simulink library "vmc"  (R2021b)
settings: Solver=VariableStepAuto  StartTime=0.0  StopTime=10.0  RelTol=1e-3
undefined symbols (not defined in the file or in its folder): AVMC_ACCDeltaTqIGain_X_kph, AVMC_ACCDeltaTqIGain_Y_mps2, AVMC_ACCDeltaTqPGain_X_kph, AVMC_ACCDeltaTqPGain_Y_kph, AVMC_ACCLongSteadyCtrl_X_kph, AVMC_AggressJerkPCT4AT_X_kph, AVMC_AggressJerkPCT_X_kph, AVMC_AggressLimitPCT4AT_X_kph, AVMC_AggressLimitPCT_X_kph, AVMC_CCLongSteadyCtrl_X_kph, AVMC_DISCDeltaTqIGain_X_kph, AVMC_DISCDeltaTqIGain_Y_mps2, AVMC_DISCDeltaTqPGain_X_kph, AVMC_DISCDeltaTqPGain_Y_kph, AVMC_DISCTrunAccJerk_X_s, AVMC_DISCTrunAccLimit_X_s, AVMC_ESCRegenOut_X_kph, AVMC_ESCRegenOut_Y_Deg, AVMC_ESCRegenOutEnSpd_X_Deg, AVMC_ISOAccLimit_X_mps, AVMC_ISODecLimit_X_mps, AVMC_ISOJerk_X_mps, AVMC_LatESCRegenOut_X_kph, AVMC_LatESCRegenOut_Y_Deg, AVMC_LongAccDeadZone_X_kph, AVMC_LongAccFiltTsforP2_X_Gps, AVMC_MCPresBaseTq_X_bar, AVMC_MSALongSteadyCtrl_X_kph, AVMC_MSAPedalOvrd2_X_kph, AVMC_MSAPedalOvrd_X_kph, AVMC_MSASpdBand_X_kph, AVMC_MSATqDownEndTq_X_kph, AVMC_MSATqDownTime_X_kph, AVMC_OPDDisSlideRate_X_Deg, AVMC_RDCDetectTime_X_kph, AVMC_RDCDetectTime_Y_pct, AVMC_RDCEnSlideRate_X_Deg, AVMC_RearWhlTqRatio_X_Nm, AVMC_RearWhlTqRatio_Y_gps, AVMC_RearWhlTqSlipGain_X_rat, AVMC_RearWhlTqSlipGain_Y_kph, AVMC_RearWhlTqSTRGGain_X_deg, AVMC_RearWhlTqSTRGGain_Y_kph, AVMC_RWSRrTSA2RWSPos_X_deg, AVMC_RWSSAS2FrtTSA_X_deg, AVMC_RWSVehSPD2RWSCoef_X_kph, AVMC_SoftJerkPCT_X_kph, AVMC_SoftLimitPCT_X_kph, AVMC_StESCYaw_X_kph, AVMC_StESCYaw_Y_Deg, AVMC_StESCYawCom_X_kph, AVMC_StESCYawCom_Y_Gps, AVMC_TMSpdBaseTq_X_rpm, AVMC_VehHoldBDecMap_X_kph, AVMC_VehHoldDecCtrlTime_X_kph, AVMC_VehHoldMCPPass_X_deg, C_TASK_10MS_S, C_TASK_5MS_S, DEG2RAD, ENUM_ACCAVAIL_AVAILABLE ... (+409)
libraries: hcu_lib x74, simulink x68, simulink_extras x3, $bdroot x2
(part 1 of 15)
settings Model: Creator=FVT22120  LastModifiedBy=FVT23010

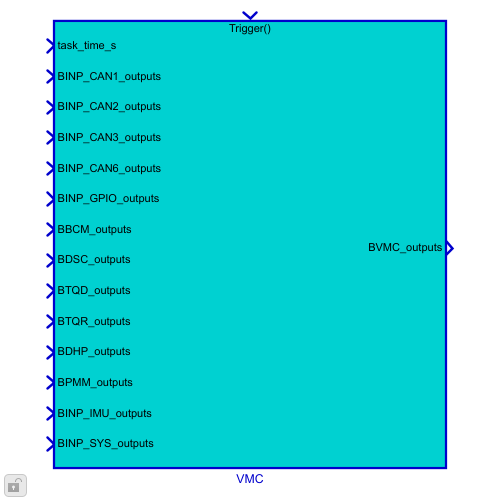
[thumbnail: Simulink's stored preview of the top-level diagram]
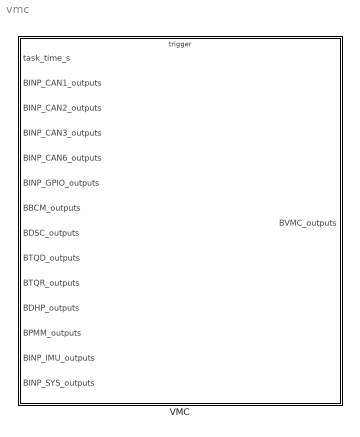
== system vmc ==
  VMC : Subsystem
      settings: RTWSystemCode=Nonreusable function  RTWFcnNameOpts=Use subsystem name  RTWFileNameOpts=Use subsystem name

== system vmc/VMC ==
  task_time_s : Inport
  BINP_CAN1_outputs : Inport  Port=2  OutDataTypeStr=Bus: BINP_CAN1_outputs
  BINP_CAN2_outputs : Inport  Port=3  OutDataTypeStr=Bus: BINP_CAN2_outputs
  BINP_CAN3_outputs : Inport  Port=4  OutDataTypeStr=Bus: BINP_CAN3_outputs
  BINP_CAN6_outputs : Inport  Port=5  OutDataTypeStr=Bus: BINP_CAN6_outputs
  BINP_GPIO_outputs : Inport  Port=6  OutDataTypeStr=Bus: BINP_GPIO_outputs
  BBCM_outputs : Inport  Port=7  OutDataTypeStr=Bus: BBCM_outputs
  BDSC_outputs : Inport  Port=8  OutDataTypeStr=Bus: BDSC_outputs
  BTQD_outputs : Inport  Port=9  OutDataTypeStr=Bus: BTQD_outputs
  BTQR_outputs : Inport  Port=10  OutDataTypeStr=Bus: BTQR_outputs
  BDHP_outputs : Inport  Port=11  OutDataTypeStr=Bus: BDHP_outputs
  BPMM_outputs : Inport  Port=12  OutDataTypeStr=Bus: BPMM_outputs
  BINP_IMU_outputs : Inport  Port=13  OutDataTypeStr=Bus: BINP_IMU_outputs
  BINP_SYS_outputs : Inport  Port=14  OutDataTypeStr=Bus: BINP_SYS_outputs
  Trigger : TriggerPort  TriggerType=function-call  VariantControl=(inherit)  PortDimensions=1
  Bus Creator1 : BusCreator  Inputs=148  OutDataTypeStr=Bus: BVMC_outputs  NonVirtualBus=on
  Bus Selector : BusSelector  OutputSignals=VINP_DriverSeatBeltCmd_flg,VINP_MeterIndVehSpeed_kph,VINP_BrkSwSta_flg,VINP_EPBSta_enum,VINP_ACCAvail_flg,VINP_AEBAvail_flg,VINP_ESCOFFStatus_enum,VINP_VehSpeed_kph,VINP_LFRawWhlSpeed_kph,VINP_LFRawWhlSpeedV_flg,VINP_RFRawWhlSpeed_kph,VINP_RFRawWhlSpeedV_flg,VINP_LRRawWhlSpeed_kph,VINP_LRRawWhlSpeedV_flg,VINP_RRRawWhlSpeed_kph,VINP_RRRawWhlSpeedV_flg,VINP_LatAccel_Gps,VINP_LatAccelV_flg,VINP_GRADE_Deg,VINP_LongAccel_Gps,VINP_MCPressure_bar,VINP_ESCADASSta_enum,VINP_FrRBCActive_flg,VINP_RrRBCActive_flg,VINP_FrntAxlTrqReqBrk_Nm,VINP_RearAxlTrqReqBrk_Nm,VINP_BrkPedalPos_pct,VINP_SASAngle_Deg,VINP_ESCActive_flg,VINP_YawRate_degps,VINP_RDCActive_enum,VINP_LFWhlRotDir_enum,VINP_LRWhlRotDir_enum,VINP_RFWhlRotDir_enum,VINP_RRWhlRotDir_enum
  Bus Selector10 : BusSelector  OutputSignals=VDHP_ActAPSPosn_pct
  Bus Selector11 : BusSelector  OutputSignals=VPMM_DrivetrainSelect_enum
  Bus Selector12 : BusSelector  OutputSignals=VINP_DIDGetDynoMode_flg
  Bus Selector2 : BusSelector  OutputSignals=VBCM_DrDoorSW_flg
  Bus Selector3 : BusSelector  OutputSignals=VDSC_DISCTurn_flg,VDSC_DISCSta_enum,VDSC_DISCTargetSpd_kph
  Bus Selector4 : BusSelector  OutputSignals=VTQD_DriverWhlTqDem_Nm,VTQD_CoordWhlTqDemFr_Nm,VTQD_CoordWhlTqDemRr_Nm,VTQD_GearActualPosn_enum,VTQD_ExternalTqAllow_flg,VTQD_LowIdleAccPedal_flg,VTQD_ExtShftAllow_flg,VTQD_FrEDUAvailBrkRgnTq_Nm,VTQD_RrEDUAvailBrkRgnTq_Nm,VTQD_APSStaSys_enum,VTQD_APSDecReqA_flg,VTQD_APSDecReq_mps2,VTQD_APSReq_enum,VTQD_AfterAvailableTqDemFr_Nm,VTQD_AfterAvailableTqDemRr_Nm,VTQD_EquivAccPedalSWSta_flg,VTQD_ExtDoorAllow_flg,VTQD_SpdCtrlSta_flg,VTQD_SpdCtrlMode_enum,VTQD_RegenMode_enum,VTQD_SetSpd_kph,VTQD_SWCResUpSta_flg,VTQD_SWCSetdownSta_flg,VTQD_SWCCancelSta_flg,VTQD_CreepBaseTqD_Nm
  Bus Selector5 : BusSelector  OutputSignals=VINP_FrTMSpd_rpm,VINP_RrTMSpd_rpm
  Bus Selector6 : BusSelector  OutputSignals=VINP_BrakeSWGPIO_flg,VINP_HoodSW_flg
  Bus Selector7 : BusSelector  OutputSignals=VINP_ADASAEBSta_enum,VINP_ADASACCSta_enum,VINP_ACCRequiredAccel_mps2,VINP_ACCVehHoldReq_flg,VINP_ADASAEBReq_enum,VINP_ADASLKASta_enum,VINP_FCMLKAStrToqReq_Nm,VINP_FCMLKATOIFault_flg,VINP_FCMLKATOIAct_enum,VINP_ADASFaultSta_flg,VINP_AEBVehHoldReq_flg,VINP_ADASDBSReq_enum,VINP_ACCObjDist_m,VINP_ACCObjRelSpd_mps,VINP_TimeGapLevel_enum,VINP_HazardWarningReq_flg,VINP_ADASForceIdle_flg,VINP_RightTurnLightReq_flg,VINP_LeftTurnLightReq_flg,VINP_ForceLowBeam_enum,VINP_ACCJerkUpperLimit_mps3,VINP_ACCComfortBandUpper_mps2,VINP_ACCJerkLowerLimit_mps3,VINP_ACCComfortBandLower_mps2,VINP_ADASVehSpdLim_enum,VINP_ADASShftPosnReqA_flg,VINP_ADASShftPosnReq_enum,VINP_ADASFCWSta_enum,VINP_ADASLDWSta_enum,VINP_ADASFltWrnReq_flg,VINP_ACCObjDstLvl_enum,VINP_ACCTakeoverReq_flg,VINP_ADASWarningMsg_enum,VINP_ADASCAMSpdLim_enum,VINP_TargetType_enum,VINP_ADASSLIFSpdLim_enum,VINP_LKAHODDisplayWarning_flg,VINP_LKAHODSoundWarning_flg,VINP_ADASLFCSta_enum,VINP_ADASLaneModeL_enum,VINP_ADASLaneModeR_enum,VINP_ADASSLIFSta_enum,VINP_ADASISASta_enum,VINP_ADASLDWMute_flg,VINP_ADASFCWMute_flg,VINP_ADASLFCHandsOffWarning_enum,VINP_LVDADisabled_flg,VINP_LVDAMuteSta_enum,VINP_LVDAFailinfo_flg,VINP_LVDAWarning_flg,VINP_LVDAACCStatusInformation_flg,VINP_ADASLFCWarnSound_enum
  Bus Selector8 : BusSelector  OutputSignals=VINP_Distanceunit_flg,VINP_METERKPHCalcu_kph,VINP_GPSLAT_s,VINP_GPSLONG_enum
  Bus Selector9 : BusSelector  OutputSignals=VTQR_RrTMTqReq_Nm,VTQR_FrTMTqReq_Nm
  Ground{,1..20} (21 alike) : Ground
  VMC : Subsystem
  BVMC_outputs : Outport  OutDataTypeStr=Bus:BVMC_outputs
  wires:
  Bus Selector/24 -> VMC/25(VINP_RrRBCActive_flg)  "<VINP_RrRBCActive_flg>"
  Bus Selector/23 -> VMC/24(VINP_FrRBCActive_flg)  "<VINP_FrRBCActive_flg>"
  BINP_CAN3_outputs/1 -> Bus Selector5/1
  Bus Selector/22 -> VMC/23(VINP_ESCADASSta_enum)  "<VINP_ESCADASSta_enum>"
  Bus Selector/21 -> VMC/22(VINP_MCPressure_bar)  "<VINP_MCPressure_bar>"
  Bus Selector7/9 -> VMC/52(VINP_LKATOIAct_enum)  "<VINP_FCMLKATOIAct_enum>"
  Bus Selector7/8 -> VMC/51(VINP_LKATOIFault_flg)  "<VINP_FCMLKATOIFault_flg>"
  Bus Selector4/7 -> VMC/127(VTQD_ExtShftAllow_flg)  "<VTQD_ExtShftAllow_flg>"
  Bus Selector4/6 -> VMC/126(VTQD_LowIdleAccPedal_flg)  "<VTQD_LowIdleAccPedal_flg>"
  Bus Selector8/1 -> VMC/37(VINP_Distanceunit_flg)  "<VINP_Distanceunit_flg>"
  Bus Selector/1 -> VMC/2(VINP_DriverSeatBeltCmd_flg)  "<VINP_DriverSeatBeltCmd_flg>"
  Bus Selector7/15 -> VMC/58(VINP_TimeGapLevel_enum)  "<VINP_TimeGapLevel_enum>"
  Bus Selector7/14 -> VMC/57(VINP_ACCObjRelSpd_mps)  "<VINP_ACCObjRelSpd_mps>"
  Bus Selector7/13 -> VMC/56(VINP_ACCObjDist_m)  "<VINP_ACCObjDist_m>"
  Bus Selector7/12 -> VMC/55(VINP_ADASDBSReq_enum)  "<VINP_ADASDBSReq_enum>"
  Bus Selector7/11 -> VMC/54(VINP_AEBVehHoldReq_flg)  "<VINP_AEBVehHoldReq_flg>"
  Bus Selector7/10 -> VMC/53(VINP_ADASFaultSta_flg)  "<VINP_ADASFaultSta_flg>"
  Bus Selector7/7 -> VMC/50(VINP_LKAStrToqReq_Nm)  "<VINP_FCMLKAStrToqReq_Nm>"
  Bus Selector7/6 -> VMC/49(VINP_ADASLKASta_enum)  "<VINP_ADASLKASta_enum>"
  Bus Selector7/5 -> VMC/48(VINP_ADASAEBReq_enum)  "<VINP_ADASAEBReq_enum>"
  Bus Selector7/4 -> VMC/47(VINP_ACCVehHoldReq_flg)  "<VINP_ACCVehHoldReq_flg>"
  Bus Selector7/3 -> VMC/46(VINP_ACCRequiredAccel_mps2)  "<VINP_ACCRequiredAccel_mps2>"
  Bus Selector7/2 -> VMC/45(VINP_ADASACCSta_enum)  "<VINP_ADASACCSta_enum>"
  Bus Selector7/1 -> VMC/44(VINP_ADASAEBSta_enum)  "<VINP_ADASAEBSta_enum>"
  BINP_CAN6_outputs/1 -> Bus Selector7/1
  Bus Selector6/1 -> VMC/101(VINP_BrakeSWGPIO_flg)  "<VINP_BrakeSWGPIO_flg>"
  BINP_GPIO_outputs/1 -> Bus Selector6/1
  task_time_s/1 -> VMC/1(task_time_s)
  Bus Selector/9 -> VMC/10(VINP_LFRawWhlSpeed_kph)  "<VINP_LFRawWhlSpeed_kph>"
  Bus Selector/10 -> VMC/11(VINP_LFRawWhlSpeedV_flg)  "<VINP_LFRawWhlSpeedV_flg>"
  Bus Selector/11 -> VMC/12(VINP_RFRawWhlSpeed_kph)  "<VINP_RFRawWhlSpeed_kph>"
  Bus Selector/12 -> VMC/13(VINP_RFRawWhlSpeedV_flg)  "<VINP_RFRawWhlSpeedV_flg>"
  Bus Selector/13 -> VMC/14(VINP_LRRawWhlSpeed_kph)  "<VINP_LRRawWhlSpeed_kph>"
  Bus Selector/14 -> VMC/15(VINP_LRRawWhlSpeedV_flg)  "<VINP_LRRawWhlSpeedV_flg>"
  Bus Selector/15 -> VMC/16(VINP_RRRawWhlSpeed_kph)  "<VINP_RRRawWhlSpeed_kph>"
  Bus Selector/16 -> VMC/17(VINP_RRRawWhlSpeedV_flg)  "<VINP_RRRawWhlSpeedV_flg>"
  Bus Selector/17 -> VMC/18(VINP_LatAccel_Gps)  "<VINP_LatAccel_Gps>"
  Bus Selector/6 -> VMC/7(VINP_AEBAvail_flg)  "<VINP_AEBAvail_flg>"
  Bus Selector/18 -> VMC/19(VINP_LatAccelV_flg)  "<VINP_LatAccelV_flg>"
  Bus Selector/5 -> VMC/6(VINP_ACCAvail_flg)  "<VINP_ACCAvail_flg>"
  Bus Selector/19 -> VMC/20(VINP_GRADE_Deg)  "<VINP_GRADE_Deg>"
  Bus Selector/2 -> VMC/3(VINP_MeterIndVehSpeed_kph)  "<VINP_MeterIndVehSpeed_kph>"
  Bus Selector4/5 -> VMC/125(VTQD_ExternalTqAllow_flg)  "<VTQD_ExternalTqAllow_flg>"
  Bus Selector4/4 -> VMC/124(VTQD_GearActualPosn_enum)  "<VTQD_GearActualPosn_enum>"
  Bus Selector4/3 -> VMC/123(VTQD_CoordWhlTqDemRr_Nm)  "<VTQD_CoordWhlTqDemRr_Nm>"
  Bus Selector4/2 -> VMC/122(VTQD_CoordWhlTqDemFr_Nm)  "<VTQD_CoordWhlTqDemFr_Nm>"
  Bus Selector4/1 -> VMC/121(VTQD_DriverWhlTqDem_Nm)  "<VTQD_DriverWhlTqDem_Nm>"
  Bus Selector/20 -> VMC/21(VINP_LongAccel_Gps)  "<VINP_LongAccel_Gps>"
  Bus Selector/7 -> VMC/8(VINP_ESCOFFStatus_enum)  "<VINP_ESCOFFStatus_enum>"
  Bus Selector/8 -> VMC/9(VINP_VehSpeed_kph)  "<VINP_VehSpeed_kph>"
  Bus Selector/4 -> VMC/5(VINP_EPBSta_enum)  "<VINP_EPBSta_enum>"
  Bus Selector/3 -> VMC/4(VINP_BrkSwSta_flg)  "<VINP_BrkSwSta_flg>"
  BTQD_outputs/1 -> Bus Selector4/1
  Bus Selector3/3 -> VMC/117(VDSC_DISCTargetSpd_kph)  "<VDSC_DISCTargetSpd_kph>"
  Bus Selector3/2 -> VMC/116(VDSC_DISCSta_enum)  "<VDSC_DISCSta_enum>"
  Bus Selector3/1 -> VMC/115(VDSC_DISCTurn_flg)  "<VDSC_DISCTurn_flg>"
  BDSC_outputs/1 -> Bus Selector3/1
  Bus Selector2/1 -> VMC/114(VBCM_DrDoorSW_flg)  "<VBCM_DrDoorSW_flg>"
  BBCM_outputs/1 -> Bus Selector2/1
  BINP_CAN1_outputs/1 -> Bus Selector/1
  Bus Creator1/1 -> BVMC_outputs/1  "BVMC_outputs"
  Bus Selector/25 -> VMC/26(VINP_FrntAxlTrqReqBrk_Nm)  "<VINP_FrntAxlTrqReqBrk_Nm>"
  Bus Selector/26 -> VMC/27(VINP_RearAxlTrqReqBrk_Nm)  "<VINP_RearAxlTrqReqBrk_Nm>"
  Bus Selector7/16 -> VMC/59(VINP_HazardWarningReq_flg)  "<VINP_HazardWarningReq_flg>"
  BTQR_outputs/1 -> Bus Selector9/1
  Bus Selector9/1 -> VMC/147(VTQR_RrTMTqReq_Nm)  "<VTQR_RrTMTqReq_Nm>"
  Bus Selector/27 -> VMC/28(VINP_BrkPedalPos_pct)  "<VINP_BrkPedalPos_pct>"
  Bus Selector4/9 -> VMC/129(VTQD_RrEDUAvailBrkRgnTq_Nm)  "<VTQD_RrEDUAvailBrkRgnTq_Nm>"
  Bus Selector4/10 -> VMC/130(VTQD_APSStaSys_enum)  "<VTQD_APSStaSys_enum>"
  Bus Selector4/11 -> VMC/131(VTQD_APSDecReqA_flg)  "<VTQD_APSDecReqA_flg>"
  Bus Selector4/12 -> VMC/132(VTQD_APSDecReq_mps2)  "<VTQD_APSDecReq_mps2>"
  Bus Selector4/13 -> VMC/133(VTQD_APSReq_enum)  "<VTQD_APSReq_enum>"
  Bus Selector4/14 -> VMC/134(VTQD_AfterAvailableTqDemFr_Nm)  "<VTQD_AfterAvailableTqDemFr_Nm>"
  Bus Selector4/15 -> VMC/135(VTQD_AfterAvailableTqDemRr_Nm)  "<VTQD_AfterAvailableTqDemRr_Nm>"
  Bus Selector4/16 -> VMC/136(VTQD_EquivAccPedalSWSta_flg)  "<VTQD_EquivAccPedalSWSta_flg>"
  BDHP_outputs/1 -> Bus Selector10/1
  Bus Selector10/1 -> VMC/149(VDHP_ActAPSPosn_pct)  "<VDHP_ActAPSPosn_pct>"
  VMC/1(VVMC_FeatSetSpdFinal_raw32) -> Bus Creator1/1
  VMC/2(VVMC_VehicleSpeed_mph) -> Bus Creator1/2
  VMC/3(VVMC_VehicleSpeed_kph) -> Bus Creator1/3
  VMC/4(VVMC_MeterIndSpeed_raw32) -> Bus Creator1/4
  VMC/5(VVMC_MeterIndSpeedForCalcu_kph) -> Bus Creator1/5
  VMC/6(VVMC_VMCAEBCtrlAvail_flg) -> Bus Creator1/6
  VMC/7(VVMC_VMCACCCtrlAvail_flg) -> Bus Creator1/7
  VMC/8(VVMC_VMCCCCtrlAvail_flg) -> Bus Creator1/8
  VMC/9(VVMC_VMCMSACtrlAvail_flg) -> Bus Creator1/9
  VMC/10(VVMC_FeatArbitrSta_enum) -> Bus Creator1/10
  VMC/11(VVMC_FeatReqSpd_kph) -> Bus Creator1/11
  VMC/12(VVMC_JerkPCT_pct) -> Bus Creator1/12
  VMC/13(VVMC_LimitPCT_pct) -> Bus Creator1/13
  VMC/14(VVMC_LFWhlSpeedRollAve_kph) -> Bus Creator1/14
  VMC/15(VVMC_RFWhlSpeedRollAve_kph) -> Bus Creator1/15
  VMC/16(VVMC_LRWhlSpeedRollAve_kph) -> Bus Creator1/16
  VMC/17(VVMC_RRWhlSpeedRollAve_kph) -> Bus Creator1/17
  VMC/18(VVMC_FrontRearSlipRatioCtrl_flg) -> Bus Creator1/18
  VMC/19(VVMC_RearWhlSlipRatioCtrl_flg) -> Bus Creator1/19
  VMC/20(VVMC_SingleWhlSlipRatioCtrl_flg) -> Bus Creator1/20
  VMC/21(VVMC_LatAccCtrl_flg) -> Bus Creator1/21
  VMC/22(VVMC_SafetyCtrl_flg) -> Bus Creator1/22
  VMC/23(VVMC_EstSlope_Deg) -> Bus Creator1/23
  VMC/24(VVMC_SPD2ACCAct_flg) -> Bus Creator1/24
  VMC/25(VVMC_AccCalcuPID_mps2) -> Bus Creator1/25
  VMC/26(VVMC_ISOAccLimit_mps2) -> Bus Creator1/26
  VMC/27(VVMC_ISODecLimit_mps2) -> Bus Creator1/27
  VMC/28(VVMC_ISOJerkLimit_mps3) -> Bus Creator1/28
  VMC/29(VVMC_ACCRequiredAccel_mps2) -> Bus Creator1/29
  VMC/30(VVMC_DISCReqAcc_mps2) -> Bus Creator1/30
  VMC/31(VVMC_FeatArbitrFinal_enum) -> Bus Creator1/31
  VMC/32(VVMC_ActACCRequiredAccel_mps2) -> Bus Creator1/32
  VMC/33(VVMC_LateralCtrl_flg) -> Bus Creator1/33
  VMC/34(VVMC_ADASLKASta_enum) -> Bus Creator1/34
  VMC/35(VVMC_LKAStrToqReq_Nm) -> Bus Creator1/35
  VMC/36(VVMC_LKATOIFault_flg) -> Bus Creator1/36
  VMC/37(VVMC_LKATOIAct_enum) -> Bus Creator1/37
  VMC/89(VVMC_ADASAEBSta_enum) -> Bus Creator1/89
  VMC/39(VVMC_ADASFaultSta_flg) -> Bus Creator1/39
  VMC/40(VVMC_AEBVehHoldReq_flg) -> Bus Creator1/40
  VMC/41(VVMC_ACCVehHoldReq_flg) -> Bus Creator1/41
  VMC/42(VVMC_ADASDBSReq_enum) -> Bus Creator1/42
  VMC/43(VVMC_ADASACCSta_enum) -> Bus Creator1/43
  VMC/44(VVMC_ACCObjDist_m) -> Bus Creator1/44
  VMC/45(VVMC_ACCObjRelSpd_mps) -> Bus Creator1/45
  VMC/46(VVMC_TimeGapLevel_enum) -> Bus Creator1/46
  VMC/47(VVMC_ACCJerkUpperLimit_mps3) -> Bus Creator1/47
  VMC/48(VVMC_ACCComfortBandUpper_mps2) -> Bus Creator1/48
  VMC/49(VVMC_ACCJerkLowerLimit_mps3) -> Bus Creator1/49
  VMC/50(VVMC_ACCComfortBandLower_mps2) -> Bus Creator1/50
  VMC/51(VVMC_ADASVehSpdLim_raw32) -> Bus Creator1/51
  VMC/52(VVMC_ADASShftPosnReqA_flg) -> Bus Creator1/52
  VMC/53(VVMC_ADASShftPosnReq_enum) -> Bus Creator1/53
  VMC/54(VVMC_ADASForceIdle_flg) -> Bus Creator1/54
  VMC/55(VVMC_HazardWarningReq_flg) -> Bus Creator1/55
  VMC/56(VVMC_RightTurnLightReq_flg) -> Bus Creator1/56
  VMC/57(VVMC_LeftTurnLightReq_flg) -> Bus Creator1/57
  VMC/58(VVMC_ADASFCWSta_enum) -> Bus Creator1/58
  VMC/59(VVMC_ADASLDWSta_enum) -> Bus Creator1/59
  VMC/60(VVMC_ADASFltWrnReq_flg) -> Bus Creator1/60
  VMC/61(VVMC_ACCObjDstLvl_enum) -> Bus Creator1/61
  VMC/62(VVMC_ForceLowBeam_enum) -> Bus Creator1/62
  VMC/63(VVMC_ACCTakeoverReq_flg) -> Bus Creator1/63
  VMC/64(VVMC_ADASWarningMsg_enum) -> Bus Creator1/64
  VMC/65(VVMC_ADASCAMSpdLim_enum) -> Bus Creator1/65
  VMC/66(VVMC_TargetType_enum) -> Bus Creator1/66
  VMC/67(VVMC_ADASSLIFSpdLim_enum) -> Bus Creator1/67
  VMC/68(VVMC_LKAHODDisplayWarning_flg) -> Bus Creator1/68
  VMC/69(VVMC_LKAHODSoundWarning_flg) -> Bus Creator1/69
  VMC/70(VVMC_ADASLFCSta_enum) -> Bus Creator1/70
  VMC/71(VVMC_ADASLaneModeL_enum) -> Bus Creator1/71
  VMC/72(VVMC_ADASLaneModeR_enum) -> Bus Creator1/72
  VMC/73(VVMC_ADASSLIFSta_enum) -> Bus Creator1/73
  VMC/74(VVMC_ADASISASta_enum) -> Bus Creator1/74
  VMC/75(VVMC_ADASLDWMute_flg) -> Bus Creator1/75
  VMC/76(VVMC_ADASFCWMute_flg) -> Bus Creator1/76
  VMC/77(VVMC_ADASLFCHandsOffWarning_enum) -> Bus Creator1/77
  VMC/78(VVMC_LVDADisabled_flg) -> Bus Creator1/78
  VMC/79(VVMC_LVDAMuteSta_enum) -> Bus Creator1/79
  VMC/80(VVMC_LVDAFailinfo_flg) -> Bus Creator1/80
  VMC/81(VVMC_LVDAWarning_flg) -> Bus Creator1/81
  VMC/82(VVMC_LVDAACCStatusInformation_flg) -> Bus Creator1/82
  VMC/83(VVMC_ADASLFCWarnSound_enum) -> Bus Creator1/83
  VMC/84(VVMC_FCMACCmode_enum) -> Bus Creator1/84
  VMC/85(VVMC_ADASLanetypeR_enum) -> Bus Creator1/85
  VMC/86(VVMC_ADASLanetypeL_enum) -> Bus Creator1/86
  VMC/87(VVMC_ADASLanecurveL_raw32) -> Bus Creator1/87
  VMC/88(VVMC_ADASLanecurveR_raw32) -> Bus Creator1/88
  VMC/38(VVMC_ADASAEBReq_enum) -> Bus Creator1/38
  VMC/90(VVMC_FCMLDWRequest_enum) -> Bus Creator1/90
  VMC/91(VVMC_FCMLDWFault_flg) -> Bus Creator1/91
  VMC/92(VVMC_ADASActive_flg) -> Bus Creator1/92
  VMC/93(VVMC_ACCCtrlAvail_flg) -> Bus Creator1/93
  VMC/94(VVMC_ADASNegReq_flg) -> Bus Creator1/94
  VMC/95(VVMC_ACCPedalOvrd_flg) -> Bus Creator1/95
  VMC/96(VVMC_ADASWhlTqReq_Nm) -> Bus Creator1/96
  VMC/97(VVMC_AccPedalOvrdDISC_flg) -> Bus Creator1/97
  VMC/98(VVMC_RearTqRatio_rat) -> Bus Creator1/98
  VMC/99(VVMC_TimeGapCalcu_s) -> Bus Creator1/99
  VMC/100(VVMC_CCCtrlSta_enum) -> Bus Creator1/100
  VMC/101(VVMC_CruzActive_flg) -> Bus Creator1/101
  VMC/102(VVMC_CCPedalOvrd_flg) -> Bus Creator1/102
  VMC/103(VVMC_CruzWhlTqReq_Nm) -> Bus Creator1/103
  VMC/104(VVMC_MSACtrlSta_enum) -> Bus Creator1/104
  VMC/105(VVMC_MSAActive_flg) -> Bus Creator1/105
  VMC/106(VVMC_MSAWhlTqReq_Nm) -> Bus Creator1/106
  VMC/107(VVMC_APSCtrlAvail_flg) -> Bus Creator1/107
  VMC/108(VVMC_APSActive_flg) -> Bus Creator1/108
  VMC/109(VVMC_APSSpeedCMD_kph) -> Bus Creator1/109
  VMC/110(VVMC_APSShiftPosnReq_enum) -> Bus Creator1/110
  VMC/111(VVMC_APSStaSys_enum) -> Bus Creator1/111
  VMC/112(VVMC_APSDecReqA_flg) -> Bus Creator1/112
  VMC/113(VVMC_APSDecReq_mps2) -> Bus Creator1/113
  VMC/114(VVMC_APSReq_enum) -> Bus Creator1/114
  VMC/115(VVMC_LongAcc_Gps) -> Bus Creator1/115
  VMC/116(VVMC_RawWhlSpdSlideRate_pct) -> Bus Creator1/116
  VMC/117(VVMC_LFWhlSpdSlideRate_pct) -> Bus Creator1/117
  VMC/118(VVMC_RFWhlSpdSlideRate_pct) -> Bus Creator1/118
  VMC/119(VVMC_LRWhlSpdSlideRate_pct) -> Bus Creator1/119
  VMC/120(VVMC_RRWhlSpdSlideRate_pct) -> Bus Creator1/120
  VMC/121(VVMC_PredictVehSpd_kph) -> Bus Creator1/121
  VMC/122(VVMC_LF4WhlSpdSlideRate_pct) -> Bus Creator1/122
  VMC/123(VVMC_RF4WhlSpdSlideRate_pct) -> Bus Creator1/123
  VMC/124(VVMC_LR4WhlSpdSlideRate_pct) -> Bus Creator1/124
  VMC/125(VVMC_RR4WhlSpdSlideRate_pct) -> Bus Creator1/125
  VMC/126(VVMC_4WhlSpdSlideRate_pct) -> Bus Creator1/126
  VMC/127(VVMC_ActMaxSlideRate_pct) -> Bus Creator1/127
  VMC/128(VVMC_ActLFSlideRate_pct) -> Bus Creator1/128
  VMC/129(VVMC_ActRFSlideRate_pct) -> Bus Creator1/129
  VMC/130(VVMC_ActLRSlideRate_pct) -> Bus Creator1/130
  VMC/131(VVMC_ActRRSlideRate_pct) -> Bus Creator1/131
  VMC/132(VVMC_AltLWhlSlideRate_pct) -> Bus Creator1/132
  VMC/133(VVMC_AltRWhlSlideRate_pct) -> Bus Creator1/133
  VMC/134(VVMC_AltWhlSlideRate_pct) -> Bus Creator1/134
  VMC/135(VVMC_CCMSASpdWar_flg) -> Bus Creator1/135
  Bus Selector9/2 -> VMC/148(VTQR_FrTMTqReq_Nm)  "<VTQR_FrTMTqReq_Nm>"
  Bus Selector4/8 -> VMC/128(VTQD_FrEDUAvailBrkRgnTq_Nm)  "<VTQD_FrEDUAvailBrkRgnTq_Nm>"
  Bus Selector7/20 -> VMC/63(VINP_ForceLowBeam_enum)  "<VINP_ForceLowBeam_enum>"
  Bus Selector7/18 -> VMC/61(VINP_RightTurnLightReq_flg)  "<VINP_RightTurnLightReq_flg>"
  Bus Selector7/19 -> VMC/62(VINP_LeftTurnLightReq_flg)  "<VINP_LeftTurnLightReq_flg>"
  Bus Selector7/17 -> VMC/60(VINP_ADASForceIdle_flg)  "<VINP_ADASForceIdle_flg>"
  Bus Selector8/2 -> VMC/38(VINP_METERKPHCalcu_kph)  "<VINP_METERKPHCalcu_kph>"
  BINP_CAN2_outputs/1 -> Bus Selector8/1
  Bus Selector7/21 -> VMC/64(VINP_ACCJerkUpperLimit_mps3)  "<VINP_ACCJerkUpperLimit_mps3>"
  Bus Selector7/22 -> VMC/65(VINP_ACCComfortBandUpper_mps2)  "<VINP_ACCComfortBandUpper_mps2>"
  Bus Selector7/23 -> VMC/66(VINP_ACCJerkLowerLimit_mps3)  "<VINP_ACCJerkLowerLimit_mps3>"
  Bus Selector7/24 -> VMC/67(VINP_ACCComfortBandLower_mps2)  "<VINP_ACCComfortBandLower_mps2>"
  Bus Selector7/25 -> VMC/68(VINP_ADASVehSpdLim_raw32)  "<VINP_ADASVehSpdLim_enum>"
  Bus Selector7/26 -> VMC/69(VINP_ADASShftPosnReqA_flg)  "<VINP_ADASShftPosnReqA_flg>"
  Bus Selector7/27 -> VMC/70(VINP_ADASShftPosnReq_enum)  "<VINP_ADASShftPosnReq_enum>"
  Bus Selector7/28 -> VMC/71(VINP_ADASFCWSta_enum)  "<VINP_ADASFCWSta_enum>"
  Bus Selector7/29 -> VMC/72(VINP_ADASLDWSta_enum)  "<VINP_ADASLDWSta_enum>"
  Bus Selector7/30 -> VMC/73(VINP_ADASFltWrnReq_flg)  "<VINP_ADASFltWrnReq_flg>"
  Bus Selector7/31 -> VMC/74(VINP_ACCObjDstLvl_enum)  "<VINP_ACCObjDstLvl_enum>"
  Bus Selector7/32 -> VMC/75(VINP_ACCTakeoverReq_flg)  "<VINP_ACCTakeoverReq_flg>"
  Bus Selector7/33 -> VMC/76(VINP_ADASWarningMsg_enum)  "<VINP_ADASWarningMsg_enum>"
  Bus Selector7/34 -> VMC/77(VINP_ADASCAMSpdLim_enum)  "<VINP_ADASCAMSpdLim_enum>"
  Bus Selector7/35 -> VMC/78(VINP_TargetType_enum)  "<VINP_TargetType_enum>"
  Bus Selector7/36 -> VMC/79(VINP_ADASSLIFSpdLim_enum)  "<VINP_ADASSLIFSpdLim_enum>"
  Bus Selector7/37 -> VMC/80(VINP_LKAHODDisplayWarning_flg)  "<VINP_LKAHODDisplayWarning_flg>"
  Bus Selector7/38 -> VMC/81(VINP_LKAHODSoundWarning_flg)  "<VINP_LKAHODSoundWarning_flg>"
  Bus Selector7/39 -> VMC/82(VINP_ADASLFCSta_enum)  "<VINP_ADASLFCSta_enum>"
  Bus Selector7/40 -> VMC/83(VINP_ADASLaneModeL_enum)  "<VINP_ADASLaneModeL_enum>"
  Bus Selector7/41 -> VMC/84(VINP_ADASLaneModeR_enum)  "<VINP_ADASLaneModeR_enum>"
  Bus Selector7/42 -> VMC/85(VINP_ADASSLIFSta_enum)  "<VINP_ADASSLIFSta_enum>"
  Bus Selector7/43 -> VMC/86(VINP_ADASISASta_enum)  "<VINP_ADASISASta_enum>"
  Bus Selector7/44 -> VMC/87(VINP_ADASLDWMute_flg)  "<VINP_ADASLDWMute_flg>"
  Bus Selector7/45 -> VMC/88(VINP_ADASFCWMute_flg)  "<VINP_ADASFCWMute_flg>"
  Bus Selector7/46 -> VMC/89(VINP_ADASLFCHandsOffWarning_enum)  "<VINP_ADASLFCHandsOffWarning_enum>"
  Bus Selector7/47 -> VMC/90(VINP_LVDADisabled_flg)  "<VINP_LVDADisabled_flg>"
  Bus Selector7/48 -> VMC/91(VINP_LVDAMuteSta_enum)  "<VINP_LVDAMuteSta_enum>"
  Bus Selector7/49 -> VMC/92(VINP_LVDAFailinfo_flg)  "<VINP_LVDAFailinfo_flg>"
  Bus Selector7/50 -> VMC/93(VINP_LVDAWarning_flg)  "<VINP_LVDAWarning_flg>"
  Bus Selector7/51 -> VMC/94(VINP_LVDAACCStatusInformation_flg)  "<VINP_LVDAACCStatusInformation_flg>"
  Bus Selector7/52 -> VMC/95(VINP_ADASLFCWarnSound_enum)  "<VINP_ADASLFCWarnSound_enum>"
  Bus Selector/28 -> VMC/29(VINP_SASAngle_Deg)  "<VINP_SASAngle_Deg>"
  BPMM_outputs/1 -> Bus Selector11/1
  Bus Selector11/1 -> VMC/150(<VPMM_DrivetrainSelect_enum>)  "<VPMM_DrivetrainSelect_enum>"
  Ground5/1 -> VMC/43(VINP_SCPSystemMode_enum)
  VMC/136(VVMC_IMUEnaCmd_flg) -> Bus Creator1/136
  VMC/137(VVMC_RWDRDCActive_enum) -> Bus Creator1/137
  Bus Selector/29 -> VMC/30(VINP_ESCActive_flg)  "<VINP_ESCActive_flg>"
  Bus Selector/30 -> VMC/31(VINP_YawRate_degps)  "<VINP_YawRate_degps>"
  Bus Selector/31 -> VMC/32(VINP_RDCActive_enum)  "<VINP_RDCActive_enum>"
  Bus Selector4/17 -> VMC/137(VTQD_ExtDoorAllow_flg)  "<VTQD_ExtDoorAllow_flg>"
  VMC/138(VVMC_MSAWhlTqActive_flg) -> Bus Creator1/138
  Bus Selector/32 -> VMC/33(VINP_LFWhlRotDir_enum)  "<VINP_LFWhlRotDir_enum>"
  Bus Selector/33 -> VMC/34(VINP_LRWhlRotDir_enum)  "<VINP_LRWhlRotDir_enum>"
  Bus Selector/34 -> VMC/35(VINP_RFWhlRotDir_enum)  "<VINP_RFWhlRotDir_enum>"
  Bus Selector/35 -> VMC/36(VINP_RRWhlRotDir_enum)  "<VINP_RRWhlRotDir_enum>"
  Bus Selector5/1 -> VMC/41(VINP_FrTMSpd_rpm)  "<VINP_FrTMSpd_rpm>"
  Bus Selector5/2 -> VMC/42(VINP_RrTMSpd_rpm)  "<VINP_RrTMSpd_rpm>"
  BINP_IMU_outputs/1 -> VMC/151(BINP_IMU_outputs)
  VMC/139(VVMC_RDCEnSlideRate_pct) -> Bus Creator1/139
  VMC/140(VVMC_ActStESCYaw_Dps) -> Bus Creator1/140
  Bus Selector6/2 -> VMC/102(VINP_HoodSW_flg)  "<VINP_HoodSW_flg>"
  Bus Selector8/3 -> VMC/39(VINP_GPSLAT_sec)  "<VINP_GPSLAT_s>"
  Bus Selector8/4 -> VMC/40(VINP_GPSLONG_sec)  "<VINP_GPSLONG_enum>"
  BINP_SYS_outputs/1 -> Bus Selector12/1
  Bus Selector12/1 -> VMC/152(VINP_DIDGetDynoMode_flg)  "<VINP_DIDGetDynoMode_flg>"
  Bus Selector4/18 -> VMC/138(VTQD_SpdCtrlSta_flg)  "<VTQD_SpdCtrlSta_flg>"
  Bus Selector4/19 -> VMC/139(VTQD_SpdCtrlMode_enum)  "<VTQD_SpdCtrlMode_enum>"
  Bus Selector4/20 -> VMC/140(VTQD_RegenMode_enum)  "<VTQD_RegenMode_enum>"
  Bus Selector4/21 -> VMC/141(VTQD_SetSpd_kph)  "<VTQD_SetSpd_kph>"
  Bus Selector4/22 -> VMC/142(VTQD_SWCResUpSta_flg)  "<VTQD_SWCResUpSta_flg>"
  Bus Selector4/23 -> VMC/143(VTQD_SWCSetdownSta_flg)  "<VTQD_SWCSetdownSta_flg>"
  Bus Selector4/24 -> VMC/144(VTQD_SWCCANCELSta_flg)  "<VTQD_SWCCancelSta_flg>"
  Bus Selector4/25 -> VMC/145(VTQD_CreepBaseTqD_Nm)  "<VTQD_CreepBaseTqD_Nm>"
  VMC/141(VVMC_ACCOvrdMemTq_Nm) -> Bus Creator1/141
  Ground1/1 -> VMC/119(VDSC_AutoTurnMode_flg)
  Ground2/1 -> VMC/118(VDSC_TurningSpdMovingflat_kph)
  Ground4/1 -> VMC/120(VDSC_AccDecResp_flg)
  Ground6/1 -> VMC/113(VINP_CAASVMCReqA_flg)
  Ground7/1 -> VMC/111(VINP_APSDecReq_mps2)
  Ground8/1 -> VMC/112(VINP_APSReq_enum)
  Ground9/1 -> VMC/110(VINP_APSDecReqA_flg)
  Ground10/1 -> VMC/109(VINP_APSStaSystem_enum)
  Ground3/1 -> VMC/103(APP_SpdLimit_flg)
  Ground14/1 -> VMC/104(APP_SpdLimit)
  Ground13/1 -> VMC/106(VAPS_APSVMCReqA_flg)
  Ground12/1 -> VMC/105(VAPS_APSStaSystem_enum)
  Ground11/1 -> VMC/107(VAPS_APSShiftPosnReq_enum)
  Ground15/1 -> VMC/108(VAPS_APSSpeedCMD_kph)
  Ground16/1 -> VMC/100(VINP_ADASLanecurveR_raw32)
  Ground17/1 -> VMC/98(VINP_ADASLanetypeL_enum)
  Ground18/1 -> VMC/99(VINP_ADASLanecurveL_raw32)
  Ground19/1 -> VMC/97(VINP_ADASLanetypeR_enum)
  Ground20/1 -> VMC/96(VINP_FCMACCmode_enum)
  VMC/142(VVMC_CAASCtrlAvail_flg) -> Bus Creator1/142
  VMC/143(VVMC_CAASActive_flg) -> Bus Creator1/143
  VMC/144(VVMC_CalibratedGyroY_Dps) -> Bus Creator1/144
  Ground/1 -> VMC/146(VTQD_VehActSpd_kph)
  VMC/145(VVMC_VMCRWSActvSta_enum) -> Bus Creator1/145
  VMC/146(VVMC_VMCRWSDfctvSta_enum) -> Bus Creator1/146
  VMC/147(VVMC_VMCRWSPositionReq_mm) -> Bus Creator1/147
  VMC/148(VVMC_VMCSteerFaultRequest_enum) -> Bus Creator1/148
